simulink model "id_map_reference_wrapper"  (R2026a)
settings: Solver=FixedStepDiscrete  StopTime=0.0005  FixedStep=5e-4
model workspace (MAT data in the model file):
  Cal_IdMap_Iq_A_f32 = Simulink.Parameter
  Cal_IdMap_Iq_A_f32.Value = [0 5 10 15 20 25 30 35 40 45 50]
  Cal_IdMap_Iq_A_f32.Complexity = 'real'
  Cal_IdMap_Iq_A_f32.Dimensions = [1 11]
  Cal_IdMap_Iq_A_f32.CoderInfo.StorageClass = 'ExportedGlobal'
  Cal_IdMap_Iq_A_f32.Description = 'Id map q-axis current breakpoints in A.'
  Cal_IdMap_Iq_A_f32.DataType = 'single'
  Cal_IdMap_Spd_rpm_f32 = Simulink.Parameter
  Cal_IdMap_Spd_rpm_f32.Value = [0 1000 2000 3000 4000 5000 6000 7000 8000 9000 10000]
  Cal_IdMap_Spd_rpm_f32.Complexity = 'real'
  Cal_IdMap_Spd_rpm_f32.Dimensions = [1 11]
  Cal_IdMap_Spd_rpm_f32.CoderInfo.StorageClass = 'ExportedGlobal'
  Cal_IdMap_Spd_rpm_f32.Description = 'Id map speed breakpoints in rpm.'
  Cal_IdMap_Spd_rpm_f32.DataType = 'single'
  Cal_IdMap_Table_A_f32 = Simulink.Parameter
  Cal_IdMap_Table_A_f32.Value = [0  0  0  0  0  0  0  0  0  0  0; 0  0  0  0  0  0  0  0  0  0  0; 0  0  0  0  0  0  0  0  0  0  0; 0  0  0  0  0  0  0  0  0  0  0; 0  0  0  0  0  0  0  0  0  0  0; 0  0  0  0  0  0  0  0  0  0  0; 0  0  0  0  0  0  0  0  0  0  0; 0  0  0  0  0  0  0  0  0  0  0; 0  0  0  0  0  0  0  0  0  0  0; 0  0  0  0  0  0  0  0  0  0  0; 0  0  0  0  0  0  0  0  0  0  0]
  Cal_IdMap_Table_A_f32.Complexity = 'real'
  Cal_IdMap_Table_A_f32.Dimensions = [11 11]
  Cal_IdMap_Table_A_f32.CoderInfo.StorageClass = 'ExportedGlobal'
  Cal_IdMap_Table_A_f32.Description = 'Id map d-axis current output table in A.'
  Cal_IdMap_Table_A_f32.DataType = 'single'
settings Model: Creator=ASUS  LastModifiedBy=ASUS
settings RTWCC: SystemTargetFile=ert.tlc  GenCodeOnly=on  GenerateMakefile=off  Description=Embedded Coder

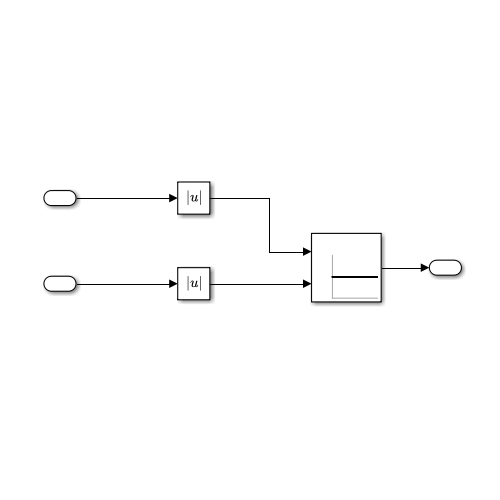
[thumbnail: Simulink's stored preview of the top-level diagram]
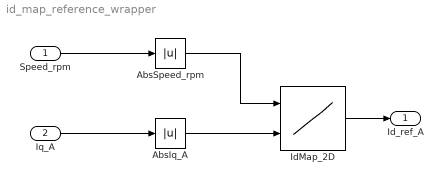
== system id_map_reference_wrapper ==
  Speed_rpm : Inport  OutDataTypeStr=single
  Iq_A : Inport  Port=2  OutDataTypeStr=single
  AbsIq_A : Abs  SaturateOnIntegerOverflow=off
  AbsSpeed_rpm : Abs  SaturateOnIntegerOverflow=off
  IdMap_2D : Lookup_n-D  LookupTableObject=''  BreakpointsForDimension1=Cal_IdMap_Spd_rpm_f32  BreakpointsForDimension2=Cal_IdMap_Iq_A_f32  BreakpointsForDimension1FirstPoint=10  BreakpointsForDimension2FirstPoint=10  BreakpointsForDimension1Spacing=12  BreakpointsForDimension2Spacing=12  Table=Cal_IdMap_Table_A_f32  TableDataTypeStr=single  IntermediateResultsDataTypeStr=single  ExtrapMethod=Clip  SampleTime=5e-4  InternalRulePriority=Speed  OutDataTypeStr=single  RndMeth=Simplest
      settings: InputPortMap=u0,u1
  Id_ref_A : Outport  OutDataTypeStr=single
  wires:
  IdMap_2D/1 -> Id_ref_A/1
  AbsIq_A/1 -> IdMap_2D/2
  AbsSpeed_rpm/1 -> IdMap_2D/1
  Iq_A/1 -> AbsIq_A/1
  Speed_rpm/1 -> AbsSpeed_rpm/1
